simulink model "respuestas_discretas"  (R2023a)
settings: Solver=VariableStepAuto  StartTime=0.0  StopTime=500  RelTol=1e-3
libraries: simulink x2, dspsrcs4 x1
settings Model: Creator=MSI  LastModifiedBy=MSI

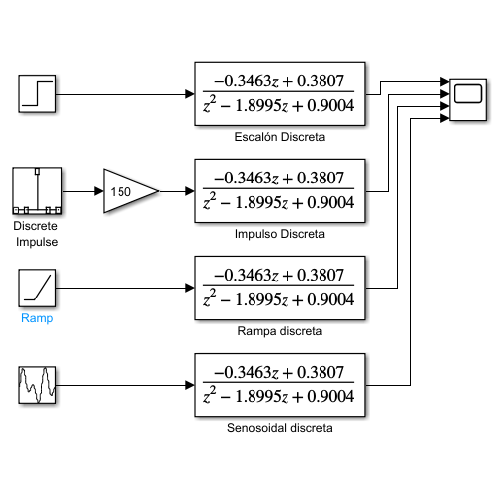
[thumbnail: Simulink's stored preview of the top-level diagram]
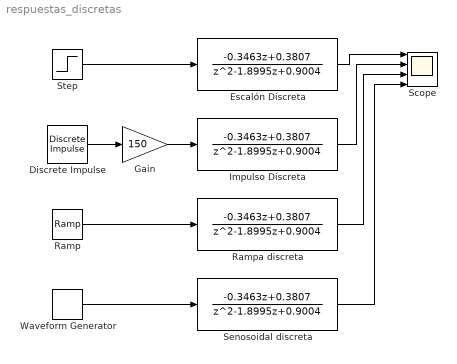
== system respuestas_discretas ==
  Discrete Impulse : dspsrcs4/Discrete  Impulse  Delay=1  SampleTime=1  FrameSample=1  OutputFrames=off  dataType=double  isSigned=on  wordLen=16  udDataType=sfix(16)  fracBitsMode=Best precision  numFracBits=15  OutDataTypeStr=double  LastOutDataTypeStr=double
  Escalón Discreta : DiscreteTransferFcn  Numerator=[0 -0.3463 0.3807]  Denominator=[1 -1.8995 0.9004]
  Gain : Gain  Gain=150
  Impulso Discreta : DiscreteTransferFcn  Numerator=[0 -0.3463 0.3807]  Denominator=[1 -1.8995 0.9004]
  Ramp : simulink/Sources/Ramp  slope=0.0025  start=0  InitialOutput=0
  Rampa discreta : DiscreteTransferFcn  Numerator=[0 -0.3463 0.3807]  Denominator=[1 -1.8995 0.9004]
  Scope : Scope  NumInputPorts=4
  Senosoidal discreta : DiscreteTransferFcn  Numerator=[0 -0.3463 0.3807]  Denominator=[1 -1.8995 0.9004]
  Step : Step  SampleTime=0
  Waveform Generator : simulink/Sources/Waveform Generator  OutMin=[]  OutMax=[]  OutDataTypeStr=double  SelectedSignal=1  Signals=sin(1,0.1,0)  BlockNames=MultiportSwitch_9682cf532b914d3  SampleTime=0.1
  wires:
  Step/1 -> Escalón Discreta/1
  Waveform Generator/1 -> Senosoidal discreta/1
  Ramp/1 -> Rampa discreta/1
  Discrete Impulse/1 -> Gain/1
  Impulso Discreta/1 -> Scope/2
  Gain/1 -> Impulso Discreta/1
  Escalón Discreta/1 -> Scope/1
  Rampa discreta/1 -> Scope/3
  Senosoidal discreta/1 -> Scope/4
